simulink model "succ_loop_whole_model"  (R2019b)
settings: Solver=VariableStepAuto  StartTime=0.0  StopTime=2000  RelTol=1e-3
values from neighbouring files (symbols this model uses):
  A = [-0.322, 0.052, 0.028, -1.12,  0.002 ... (first row only)    [oppg2f.m]
  a1 = 2.87    [oppg2c.m]    (also in oppg2e.m; oppg2f.m)
  a2 = -0.65    [oppg2c.m]    (also in oppg2e.m; oppg2f.m)
  B = [0,0,0,0,7.5]'    [oppg2f.m]
  dist = 1.5    [oppg2e.m]    (also in oppg2f.m)
  g = 9.81    [oppg2e.m]    (also in oppg2f.m)
  Kd_phi = 1.935    [oppg2e.m]    (also in oppg2f.m)
  Ki_phi = 0    [oppg2e.m]    (also in oppg2f.m)
  Ki_x = omega_n_x^2 *Vg/g    (= 0.213420550459)    [oppg2e.m]    (also in oppg2f.m)
  Kp_phi = -2    [oppg2e.m]    (also in oppg2f.m)
  Kp_x = 2*zeta_x*omega_n_x*Vg/g    (= 7.48844036697)    [oppg2e.m]    (also in oppg2f.m)
  Vg = 161.1    [oppg2e.m]    (also in oppg2f.m)
settings Model: Creator=jacob  LastModifiedBy=jacob

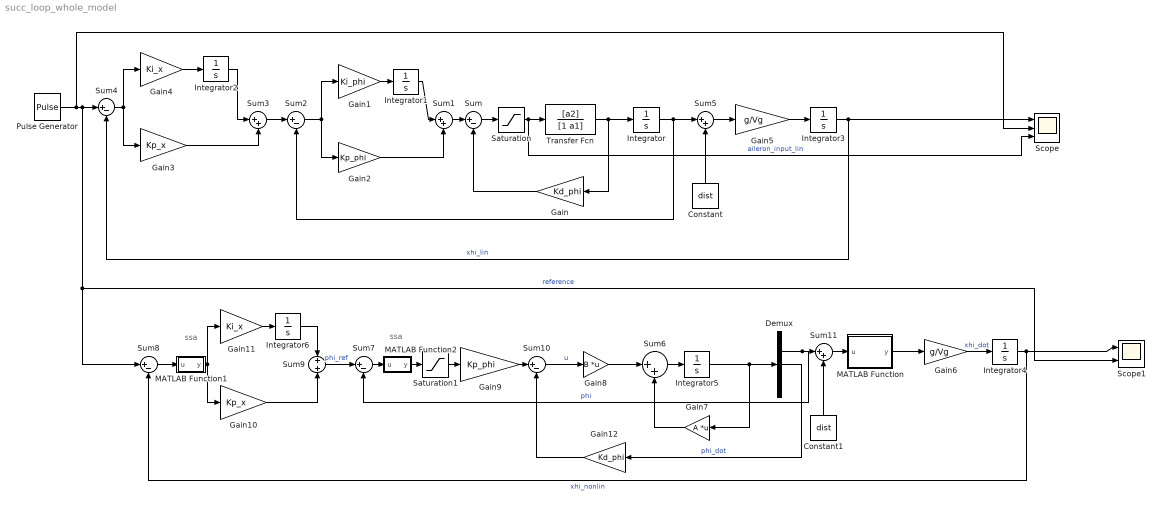
== system succ_loop_whole_model ==
  note: ssa
  note: ssa
  Constant : Constant  Value=dist
  Constant1 : Constant  Value=dist
  Demux : Demux  Outputs=5
  Gain : Gain  Gain=Kd_phi
  Gain1 : Gain  Gain=Ki_phi
  Gain10 : Gain  Gain=Kp_x
  Gain11 : Gain  Gain=Ki_x
  Gain12 : Gain  Gain=Kd_phi
  Gain2 : Gain  Gain=Kp_phi
  Gain3 : Gain  Gain=Kp_x
  Gain4 : Gain  Gain=Ki_x
  Gain5 : Gain  Gain=g/Vg
  Gain6 : Gain  Gain=g/Vg
  Gain7 : Gain  Gain=A  Multiplication=Matrix(K*u)
  Gain8 : Gain  Gain=B  Multiplication=Matrix(K*u)
  Gain9 : Gain  Gain=Kp_phi
  Integrator{,1..4,6} (6 alike) : Integrator
  Integrator5 : Integrator  InitialCondition=[0,0,0,0,0]
  MATLAB Function : MATLAB Function  TreatAsAtomicUnit=on
  MATLAB Function1 : MATLAB Function  TreatAsAtomicUnit=on
  MATLAB Function2 : MATLAB Function  TreatAsAtomicUnit=on
  Pulse Generator : DiscretePulseGenerator  PulseType=Time based  Amplitude=10  Period=400  PulseWidth=50
  Saturation : Saturate  UpperLimit=30  LowerLimit=-30
  Saturation1 : Saturate  UpperLimit=15  LowerLimit=-15
  Scope : Scope  NumInputPorts=3
  Scope1 : Scope  NumInputPorts=2
  Sum{,2,4,7..8,10} (6 alike) : Sum  Inputs=|+-
  Sum{1,3,5..6,11} (5 alike) : Sum  Inputs=|++
  Sum9 : Sum
  Transfer Fcn : TransferFcn  Numerator=[a2]  Denominator=[1 a1]
  wires:
  Transfer Fcn/1 -> Integrator/1, Gain/1
  Gain5/1 -> Integrator3/1
  Sum5/1 -> Gain5/1
  Sum3/1 -> Sum2/1
  Gain3/1 -> Sum3/2
  Integrator2/1 -> Sum3/1
  Sum/1 -> Saturation/1
  Integrator1/1 -> Sum1/1
  Gain1/1 -> Integrator1/1
  Sum2/1 -> Gain2/1, Gain1/1
  Gain4/1 -> Integrator2/1
  Constant/1 -> Sum5/2
  Sum1/1 -> Sum/1
  Sum4/1 -> Gain3/1, Gain4/1
  Pulse Generator/1 -> Scope/2, Scope1/2, Sum8/1, Sum4/1  "reference"
  Gain2/1 -> Sum1/2
  Gain/1 -> Sum/2
  Saturation/1 -> Scope/3, Transfer Fcn/1  "aileron_input_lin"
  Integrator3/1 -> Sum4/2, Scope/1  "xhi_lin"
  Integrator/1 -> Sum2/2, Sum5/1
  Gain6/1 -> Integrator4/1  "xhi_dot"
  Integrator4/1 -> Scope1/1, Sum8/2  "xhi_nonlin"
  Demux/2 -> Sum7/2, Sum11/1  "phi"
  Integrator5/1 -> Demux/1, Gain7/1
  Gain11/1 -> Integrator6/1
  Integrator6/1 -> Sum9/1
  Gain10/1 -> Sum9/2
  Sum6/1 -> Integrator5/1
  Gain7/1 -> Sum6/2
  Gain8/1 -> Sum6/1
  Gain12/1 -> Sum10/2
  Gain9/1 -> Sum10/1
  Sum9/1 -> Sum7/1  "phi_ref"
  Demux/3 -> Gain12/1  "phi_dot"
  MATLAB Function/1(y) -> Gain6/1
  Sum8/1 -> MATLAB Function1/1(u)
  MATLAB Function1/1(y) -> Gain11/1, Gain10/1
  Sum7/1 -> MATLAB Function2/1(u)
  MATLAB Function2/1(y) -> Saturation1/1
  Saturation1/1 -> Gain9/1
  Sum10/1 -> Gain8/1  "u"
  Sum11/1 -> MATLAB Function/1(u)
  Constant1/1 -> Sum11/2

== matlab function succ_loop_whole_model/MATLAB Function1 ==
  data: u input; y output
function y = fcn(u)

y = ssa(u,'deg');

== matlab function succ_loop_whole_model/MATLAB Function ==
  data: u input; y output
function y = tan_deg(u)

y = tand(u);

== matlab function succ_loop_whole_model/MATLAB Function2 ==
  data: u input; y output
function y = fcn(u)

y = ssa(u,'deg');
